simulink model "poremecaj"  (R2022b)
settings: Solver=VariableStepAuto  StartTime=0.0  StopTime=600.0  RelTol=1e-3
values from neighbouring files (symbols this model uses):
  Kd_kapa_d = Kp_d*Td_d/Ku_kapa_d    (= 10.9347)    [Parametri.m]
  Kd_kapa_d_2 = 56.667    [Parametri.m]
  Ki_d = Kp_d/Ti_d/Ku_kapa_d    (= 2.21372328459)    [Parametri.m]
  Kkr_d = 123    [Parametri.m]
  Kp_d = 0.6*Kkr_d    (= 73.8)    [Parametri.m]
  Kp_kapa_1_d = Kp_d/Ku_kapa_1_d    (= 4.92)    [Parametri.m]
  Kp_kapa_d = Kp_d/Ku_kapa_d    (= 9.84)    [Parametri.m]
  Kp_kapa_d_2 = 5.3947    [Parametri.m]
  Ku_kapa_1_d = 15    [Parametri.m]
  Ku_kapa_d = 7.5    [Parametri.m]
  Ku_kapa_d_2 = 1.5    [Parametri.m]
  Td_d = Tkr_d/8    (= 1.11125)    [Parametri.m]
  Ti_d = Tkr_d/2    (= 4.445)    [Parametri.m]
libraries: fuzblock x4
settings Model: Creator=nd190052d  LastModifiedBy=nd190052d

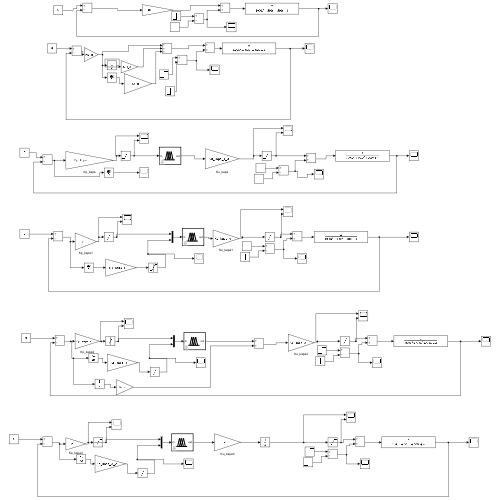
[thumbnail: Simulink's stored preview of the top-level diagram]
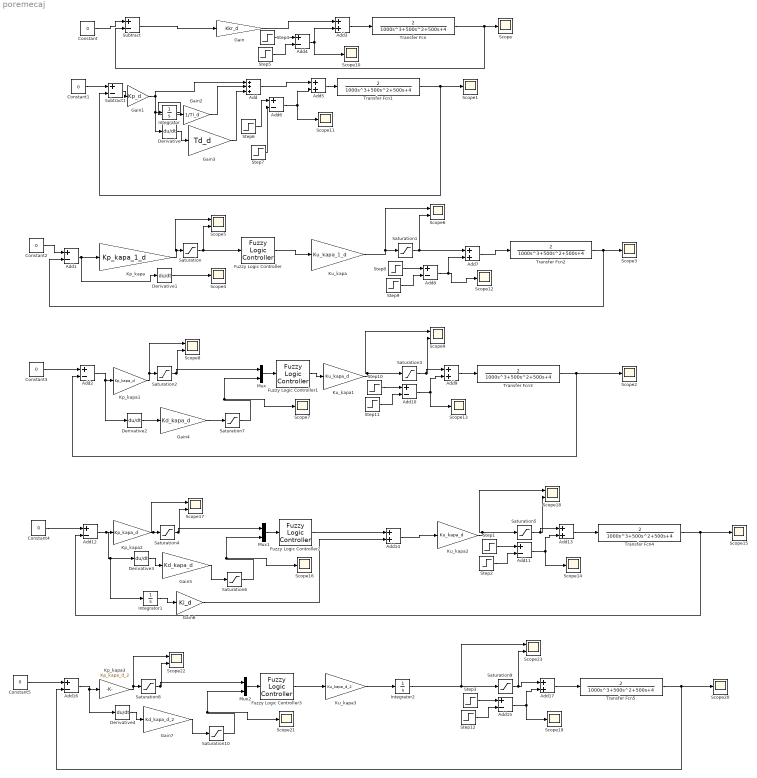
== system poremecaj ==
  Add : Sum  Inputs=+++
  Add{1..2,4,6,8,10..12,15..16} (10 alike) : Sum  Inputs=+-
  Add{3,5,7,9,13..14,17} (7 alike) : Sum
  Constant{,1..5} (6 alike) : Constant  Value=0
  Derivative{,1..4} (5 alike) : Derivative
  Fuzzy Logic Controller : fuzblock/Fuzzy Logic  Controller  FIS='sugenoP.fis'  OutputSampleNumber=101  DataType=double  FuzzifiedInputs=off  RuleFiringStrengths=off  RuleOutputs=off  AggregatedOutputs=off  SimulateUsing=Interpreted execution  OutOfRangeInputValueMessage=warning  NoRuleFiredMessage=warning  EmptyOutputFuzzySetMessage=warning
  Fuzzy Logic Controller1 : fuzblock/Fuzzy Logic  Controller  FIS='sugenoPIDnelin.fis'  OutputSampleNumber=101  DataType=double  FuzzifiedInputs=off  RuleFiringStrengths=off  RuleOutputs=off  AggregatedOutputs=off  SimulateUsing=Interpreted execution  OutOfRangeInputValueMessage=warning  NoRuleFiredMessage=warning  EmptyOutputFuzzySetMessage=warning
  Fuzzy Logic Controller2 : fuzblock/Fuzzy Logic  Controller  FIS='sugenoPIDnelin.fis'  OutputSampleNumber=101  DataType=double  FuzzifiedInputs=off  RuleFiringStrengths=off  RuleOutputs=off  AggregatedOutputs=off  SimulateUsing=Interpreted execution  OutOfRangeInputValueMessage=warning  NoRuleFiredMessage=warning  EmptyOutputFuzzySetMessage=warning
  Fuzzy Logic Controller3 : fuzblock/Fuzzy Logic  Controller  FIS='sugenoPIDnelin.fis'  OutputSampleNumber=101  DataType=double  FuzzifiedInputs=off  RuleFiringStrengths=off  RuleOutputs=off  AggregatedOutputs=off  SimulateUsing=Interpreted execution  OutOfRangeInputValueMessage=warning  NoRuleFiredMessage=warning  EmptyOutputFuzzySetMessage=warning
  Gain : Gain  Gain=Kkr_d
  Gain1 : Gain  Gain=Kp_d
  Gain2 : Gain  Gain=1/Ti_d
  Gain3 : Gain  Gain=Td_d
  Gain4 : Gain  Gain=Kd_kapa_d
  Gain5 : Gain  Gain=Kd_kapa_d
  Gain6 : Gain  Gain=Ki_d
  Gain7 : Gain  Gain=Kd_kapa_d_2
  Integrator : Integrator
  Integrator1 : Integrator
  Integrator2 : Integrator
  Kp_kapa : Gain  Gain=Kp_kapa_1_d
  Kp_kapa1 : Gain  Gain=Kp_kapa_d
  Kp_kapa2 : Gain  Gain=Kp_kapa_d
  Kp_kapa3 : Gain  Gain=Kp_kapa_d_2
  Ku_kapa : Gain  Gain=Ku_kapa_1_d
  Ku_kapa1 : Gain  Gain=Ku_kapa_d
  Ku_kapa2 : Gain  Gain=Ku_kapa_d
  Ku_kapa3 : Gain  Gain=Ku_kapa_d_2
  Mux : Mux  Inputs=2
  Mux1 : Mux  Inputs=2
  Mux2 : Mux  Inputs=2
  Saturation{,2,4,6..8,10} (7 alike) : Saturate  UpperLimit=1  LowerLimit=-1
  Saturation{1,3,5,9} (4 alike) : Saturate  UpperLimit=15  LowerLimit=-15
  Scope{,1..4,7,10..16,19..21} (16 alike) : Scope
  Scope{5..6,8..9,17..18,22..23} (8 alike) : Scope  NumInputPorts=2
  Step{1,3..4,6,8,10} (6 alike) : Step  Time=20  After=7.5  SampleTime=0
  Step{2,5,7,9,11..12} (6 alike) : Step  Time=200  After=15  SampleTime=0
  Subtract : Sum  Inputs=+-
  Subtract1 : Sum  Inputs=+-
  Transfer Fcn{,1..5} (6 alike) : TransferFcn  Numerator=[2]  Denominator=[1000 500 500 4]
  wires:
  Transfer Fcn2/1 -> Add1/2, Scope3/1
  Transfer Fcn1/1 -> Subtract1/2, Scope1/1
  Constant3/1 -> Add2/1
  Saturation/1 -> Scope5/2, Fuzzy Logic Controller/1
  Gain4/1 -> Saturation7/1
  Transfer Fcn/1 -> Subtract/2, Scope/1
  Gain3/1 -> Add/3
  Kp_kapa1/1 -> Scope8/1, Saturation2/1
  Add2/1 -> Derivative2/1, Kp_kapa1/1
  Saturation2/1 -> Mux/1, Scope8/2
  Mux/1 -> Fuzzy Logic Controller1/1
  Kp_kapa/1 -> Scope5/1, Saturation/1
  Derivative2/1 -> Gain4/1
  Ku_kapa1/1 -> Scope9/1, Saturation3/1
  Gain2/1 -> Add/2
  Ku_kapa/1 -> Scope6/1, Saturation1/1
  Derivative/1 -> Gain3/1
  Saturation3/1 -> Add9/1, Scope9/2
  Add1/1 -> Derivative1/1, Kp_kapa/1
  Gain1/1 -> Add/1, Derivative/1, Integrator/1
  Fuzzy Logic Controller1/1 -> Ku_kapa1/1
  Fuzzy Logic Controller/1 -> Ku_kapa/1
  Saturation7/1 -> Mux/2, Scope7/1
  Subtract/1 -> Gain/1
  Derivative1/1 -> Scope4/1
  Saturation1/1 -> Add7/1, Scope6/2
  Transfer Fcn3/1 -> Add2/2, Scope2/1
  Constant/1 -> Subtract/1
  Integrator/1 -> Gain2/1
  Subtract1/1 -> Gain1/1
  Add3/1 -> Transfer Fcn/1
  Gain/1 -> Add3/1
  Add4/1 -> Scope10/1, Add3/2
  Step4/1 -> Add4/1
  Step5/1 -> Add4/2
  Step7/1 -> Add6/2
  Step6/1 -> Add6/1
  Add6/1 -> Scope11/1, Add5/2
  Add5/1 -> Transfer Fcn1/1
  Add/1 -> Add5/1
  Step9/1 -> Add8/2
  Step8/1 -> Add8/1
  Add8/1 -> Add7/2, Scope12/1
  Add7/1 -> Transfer Fcn2/1
  Step11/1 -> Add10/2
  Step10/1 -> Add10/1
  Add10/1 -> Scope13/1, Add9/2
  Add9/1 -> Transfer Fcn3/1
  Constant1/1 -> Subtract1/1
  Constant2/1 -> Add1/1
  Add11/1 -> Scope14/1, Add13/2
  Step1/1 -> Add11/1
  Add13/1 -> Transfer Fcn4/1
  Constant4/1 -> Add12/1
  Add12/1 -> Integrator1/1, Derivative3/1, Kp_kapa2/1
  Step2/1 -> Add11/2
  Saturation6/1 -> Mux1/2, Scope16/1
  Saturation5/1 -> Add13/1, Scope18/2
  Transfer Fcn4/1 -> Add12/2, Scope15/1
  Saturation4/1 -> Mux1/1, Scope17/2
  Kp_kapa2/1 -> Scope17/1, Saturation4/1
  Derivative3/1 -> Gain5/1
  Gain5/1 -> Saturation6/1
  Ku_kapa2/1 -> Scope18/1, Saturation5/1
  Mux1/1 -> Fuzzy Logic Controller2/1
  Integrator1/1 -> Gain6/1
  Gain6/1 -> Add14/2
  Add14/1 -> Ku_kapa2/1
  Fuzzy Logic Controller2/1 -> Add14/1
  Transfer Fcn5/1 -> Add16/2, Scope20/1
  Saturation8/1 -> Mux2/1, Scope22/2
  Kp_kapa3/1 -> Scope22/1, Saturation8/1
  Gain7/1 -> Saturation10/1
  Saturation10/1 -> Mux2/2, Scope21/1
  Mux2/1 -> Fuzzy Logic Controller3/1
  Add15/1 -> Scope19/1, Add17/2
  Saturation9/1 -> Add17/1, Scope23/2
  Constant5/1 -> Add16/1
  Derivative4/1 -> Gain7/1
  Add17/1 -> Transfer Fcn5/1
  Step3/1 -> Add15/1
  Add16/1 -> Derivative4/1, Kp_kapa3/1
  Step12/1 -> Add15/2
  Integrator2/1 -> Saturation9/1, Scope23/1
  Fuzzy Logic Controller3/1 -> Ku_kapa3/1
  Ku_kapa3/1 -> Integrator2/1
